simulink subsystem "Biblioteca_Iconos"  (R2023a)
settings: Solver=VariableStepAuto  StartTime=0.0  StopTime=10.0  RelTol=1e-3
undefined symbols (not defined in the file): baseRobot, baseRobot_, CdG, color, Icono, M, MdI, q0_, TabAje, X, Y, Z
libraries: sm_lib x1858, nesl_utility x164
(part 1 of 39)
settings Model: Creator=albher  LastModifiedBy=albher
settings SolverCC: AlgebraicLoopSolver=TrustRegion
settings DebuggingCC: UnconnectedInputMsg=warning  UnconnectedOutputMsg=warning  UnconnectedLineMsg=warning
settings ModelReferenceCC: EnableRefExpFcnMdlSchedulingChecks=on
settings RTWCC: DLArmComputeVersion=19.05

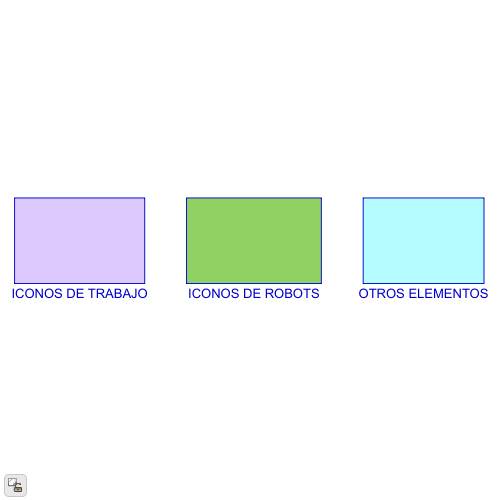
[thumbnail: Simulink's stored preview of the top-level diagram]
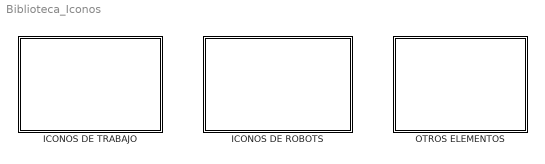
== system Biblioteca_Iconos ==
  ICONOS DE ROBOTS : Subsystem
  ICONOS DE TRABAJO : Subsystem
  OTROS ELEMENTOS : Subsystem

== system Biblioteca_Iconos/ICONOS DE ROBOTS ==
  note: image(imread(['auxStl/',tool.vNombre,'.png']))
  AbbIrb120_T_q : Subsystem  mask{base=baseRobot, q0=q0_}
      mask prompts: base "Base (x,y,z,Rz,Ry,Rx)"
      mask Display: image(imread('Robots/ABB_Irb120/AbbIrb120.png'))
  BrazoRobot : Subsystem  mask{base=baseRobot, q0=q0_}
      mask prompts: base "Base (x,y,z,Rz,Ry,Rx)"
      mask Display: image(imread('Robots/Rob_BrazoRobot/BrazoRobot.png'))
  Gofa : Subsystem  mask{base=baseRobot, q0=q0_}
      mask prompts: base "Base (x,y,z,Rz,Ry,Rx)"
      mask Display: image(imread('Robots/ABB_Gofa/abbGofa.png'))
  Humanoide : Subsystem  mask{base=baseRobot, q0=q0_}
      mask prompts: base "Base (x,y,z,Rz,Ry,Rx)"
      mask Display: image(imread('Robots/HUM_humanoide/humanoide.png'))
  Humanoide Brazos : Subsystem  mask{base=baseRobot, q0=q0_}
      mask prompts: base "Base (x,y,z,Rz,Ry,Rx)"
      mask Display: image(imread('Robots/HUM_humanoide/humanoide.png'))
  Humanoide de Pie : Subsystem  mask{base=baseRobot_, q0=q0_}
      mask prompts: base "Base (x,y,z,Rz,Ry,Rx)"
      mask Display: image(imread('Robots/HUM_humanoide/humanoide.png'))
  Niryo_Ned : Subsystem  mask{base=baseRobot, q0=q0_}
      mask prompts: base "Base(x,y,z,Rz,Ry,Rx)"
      mask Display: image(imread('Robots/NIRYO_niryo_ned/niryo_ned.png'))
  Poppy : Subsystem  mask{base=baseRobot, q0=q0_}
      mask prompts: base "Base (x,y,z,Rz,Ry,Rx)"
      mask Display: image(imread('./Robots/Poppy/Poppy.png'))
  TX40DH (q) : Subsystem  mask{base=baseRobot_, q0=q0_}
      mask prompts: base "Base [x,y,z,Rz,Ry,Rx]"
      mask init:
      | % DH de los ejes 1-6 no base
      | DH= [0, -pi/2, pi, 0, 0, 0;
      |      0.32, 0.035, 0, 0.225, 0, 0.065;
      |      0, 0.255, 0, 0, 0, 0;
      |      -pi/2, 0, pi/2, -pi/2, pi/2, 0];
      |  
      | % Sin incluir la base 
      | M= [10.8, 5.4, 4.05, 3.24, 2.16, 1.36];
      | 
      | CdG= [0, 0, 0, 0, 0, 0;
      |       0,  0, 0, 0, 0.05, 0;
      |       0.15, 0.2, 0, 0.05, 0, 0.03];
      | 
      |          % Ixx Iyy Izz Ixy Iyz Ixz
      | 
      | I=[0   ,    0.35,	0   ,	0,  0,	0;
      |    0.13 ,   0.524,	0.539,	0,	0,	0;
      |    0.066 ,  0.086,	0.0125,	0,	0,	0;
      |    0.0018,	0.0013,	0.0018,	0,	0,	0;
      |    3e-4,	4e-4,	3e-4,	0,	0,	0;
      |    1.5e-4,	1.5e-4,	4e-5,	0,	0,	0];
      | 
      | 
      | 
      | %limites
      | limits=[-pi, pi;  %Axis 1, minimum, maximum
      |         -2.18, 2.18;  %Axis 2, minimum, maximum
      |          -2.41, 2.41;   %Axis 3, minimum, maximum
      |         -4.71, 4.71;  %Axis 4, minimum, maximum
      |         -2.09, 2.09;  %Axis 5, minimum, maximum
      |         -4.71, 4.71]; %Axis 6, minimum, maximum
      |          
      | color= [1, 0.9, 0.15, 1];
      mask Display: image(imread('Robots/TX40/TX40.png'))
  "Tx90DH (q) " : Subsystem  mask{base=baseRobot_, q0=q0_}
      mask prompts: base "Base [x,y,z,Rz,Ry,Rx]"
      mask init:
      | % DH de los ejes 1-6 no base
      | DH= [0, -pi/2, pi, 0, 0, 0;
      |      0.478, 0.05, 0, 0.425, 0, 0.1;
      |      0.05, 0.425, 0, 0, 0, 0;
      |      -pi/2, 0, pi/2, -pi/2, pi/2, 0];
      |  
      | % Sin incluir la base 
      | M= [34.73, 39.27, 15.13, 21.25, 0.42, 0.03];
      | 
      | CdG= [-0.13, 0, 0.05, 0, 0.01, 0;
      |       0.47,  0, -0.55, 0.004, 0, 0;
      |       -0.18, 0, -0.14, 0, 0, 0];
      | 
      |          % Ixx Iyy Izz Ixy Iyz Ixz
      | I=[0   ,    0.35,	0   ,	0,  0,	0;
      |    0.13 ,   0.524,	0.539,	0,	0,	0;
      |    0.066 ,  0.086,	0.0125,	0,	0,	0;
      |    0.0018,	0.0013,	0.0018,	0,	0,	0;
      |    3e-4,	4e-4,	3e-4,	0,	0,	0;
      |    1.5e-4,	1.5e-4,	4e-5,	0,	0,	0];
      | 
      | %limites
      | limits=[-pi, pi;  %Axis 1, minimum, maximum
      |         -2.27, 2.57;  %Axis 2, minimum, maximum
      |         -2.53, 2.53;   %Axis 3, minimum, maximum
      |         -4.71, 4.71;  %Axis 4, minimum, maximum
      |         -2.007, 2.443;  %Axis 5, minimum, maximum
      |         -4.71, 4.71]; %Axis 6, minimum, maximum
      |          
      | color= [1, 0.4, 0.5, 1];
      mask Display: image(imread('Robots/TX90/TX90.png'))
  UR10_DH : Subsystem  mask{base=baseRobot_, q0=q0_}
      mask prompts: base "Base [x,y,z,Rz,Ry,Rx]"
      mask init:
      | % DH de los ejes 1-6 no base
      | DH= [0, pi/2, 0, -pi/2, 0, 0;
      |      0.128, 0.176, -0.128, 0.116, 0.116, 0.092;
      |      0, 0.612, 0.572, 0, 0, 0;
      |      pi/2, 0, 0, -pi/2, pi/2, 0];
      |  
      | % Sin incluir la base 
      | M= [25, 27, 15, 10, 2.5, 1.5];
      | 
      | CdG= [0, -0.05, -0.0203, 0, 0, 0;
      |       0,  0.006, -0.0141, 0.019, 0, 0;
      |       0, 0.1, 0.070, 0, 0, 0.032];
      | 
      |          % Ixx Iyy Izz Ixy Iyz Ixz
      | I=[0   ,    0.35,	0   ,	0,  0,	0;
      |    0.13 ,   0.524,	0.539,	0,	0,	0;
      |    0.066 ,  0.086,	0.0125,	0,	0,	0;
      |    0.0018,	0.0013,	0.0018,	0,	0,	0;
      |    3e-4,	4e-4,	3e-3,	0,	0,	0;
      |    1.5e-4,	1.5e-4,	4e-3,	0,	0,	0];
      | 
      | %limites
      | limits=[-pi, pi;  %Axis 1, minimum, maximum
      |         -1.74, 1.74;  %Axis 2, minimum, maximum
      |          -3.84, 3.84;   %Axis 3, minimum, maximum
      |         -3.49, 3.49;  %Axis 4, minimum, maximum
      |         -2.09, 2.09;  %Axis 5, minimum, maximum
      |         -6.98, 6.98]; %Axis 6, minimum, maximum
      |          
      | color= [0.4, 0.4, 0.6, 1];
      mask Display: image(imread('Robots/UR_UR10_DH/UR10.png'))
  gripper_3f : Subsystem  mask{base=baseRobot, q0=q0_}
      mask prompts: base "Base (x,y,z,Rz,Ry,Rx)"
      mask Display: image(imread('./Robots/gripper_3f/gripper_3f.png'))
  irb120 : Subsystem  mask{base=baseRobot, q0=q0_}
      mask prompts: base "Base (x,y,z,Rz,Ry,Rx)"
      mask Display: image(imread('Robots/ABB_irb120/AbbIrb120.png'))
  irb120_DH : Subsystem  mask{base=baseRobot, q0=q0_}
      mask prompts: base "Base [x,y,z,Rz,Ry,Rx]"
      mask init:
      | % DH de los ejes 1-6 no base
      | DH= [0, -pi/2, 0, 0, 0, pi;
      |      0.290, 0, 0, 0.302, 0, 0.072;
      |      0, 0.270, 0.070, 0, 0, 0;
      |      -pi/2, 0, -pi/2, pi/2, -pi/2, 0];
      | % Dinámica del sistema. Includo la base
      | M= 1*ones(1,7);
      | CdG= zeros(3,7);
      | MdI= 0.01*ones(6,7);
      | color= [1, 0.43, 0, 1];
      | 
      | % Límite de los ejes (rad)
      | Lim= [-165, -110, -110, -160, -120, -400;
      |       165,   110,  70,   160,  120,  400]*pi/180;
      mask Display: image(imread('Robots/ABB_irb120_DH/irb120DH.png'))
  kinovaJaco : Subsystem  mask{base=baseRobot, q0=q0_}
      mask prompts: base "Base(x,y,z,Rz,Ry,Rx)"
      mask Display: image(imread('Robots/KIN_kinova2Arm/kinovaJaco.png'))
  "puma560_DH " : Subsystem  mask{base=baseRobot, q0=q0_}
      mask prompts: base "Base [x,y,z,Rz,Ry,Rx]"
      mask init:
      | % DH de los ejes 1-6 no base
      | DH= [0, 0, 0, 0, 0, 0;
      |      0, 0, 0.15005, 0.4318, 0, 0.0;
      |      0, 0.4318, 0.0203, 0, 0, 0;
      |      pi/2, 0, -pi/2, pi/2, -pi/2, 0];
      |  
      | % Sin incluir la base 
      | M= [0, 17.4, 4.8, 0.82, 0.34, 0.09];
      | 
      | CdG= [0, -0.3638, -0.0203, 0, 0, 0;
      |       0,  0.006, -0.0141, 0.019, 0, 0;
      |       0, 0.2275, 0.070, 0, 0, 0];
      | 
      |          % Ixx Iyy Izz Ixy Iyz Ixz
      | I=[0   ,    0.35,	0   ,	0,  0,	0;
      |    0.13 ,   0.524,	0.539,	0,	0,	0;
      |    0.066 ,  0.086,	0.0125,	0,	0,	0;
      |    0.0018,	0.0013,	0.0018,	0,	0,	0;
      |    3e-4,	4e-4,	3e-4,	0,	0,	0;
      |    1.5e-4,	1.5e-4,	4e-5,	0,	0,	0];
      | 
      | %limites
      | limits=[-2.79, 2.79;  %Axis 1, minimum, maximum
      |         -1.92, 1.92;  %Axis 2, minimum, maximum
      |          -2.356, 2.356;   %Axis 3, minimum, maximum
      |         -4.642, 4.642;  %Axis 4, minimum, maximum
      |         -1.745, 1.745;  %Axis 5, minimum, maximum
      |         -4.642, 4.642]; %Axis 6, minimum, maximum
      |          
      | color= [0.4, 0.8, 0.51, 1];
      mask Display: image(imread('Robots/UNI_puma560_DH/puma560.png'))
  sawyerDH (q) : Subsystem  mask{base=baseRobot, q0=q0_}
      mask prompts: base "Base [x,y,z,Rz,Ry,Rx]"
      mask init:
      | % DH de los ejes 1-6 no base
      | DH= [0, -pi/2, 0, 0, 0, 0, 0;
      |      0.317, 0.1925, 0.4, -0.1685, 0.4, 0.1363, 0.13375;
      |      0.081, 0.0, 0.0, 0.0, 0, 0, 0;
      |      -pi/2, -pi/2, pi/2, -pi/2, pi/2, -pi/2, 0];
      |  
      | % Sin incluir la base 
      | M= [25, 27, 15, 10, 2.5,1.5, 0.09];
      | 
      | CdG= [0, -0.05, -0.0203, 0, 0, 0,0;
      |       0,  0.006, -0.0141, 0.019, 0, 0,0;
      |       0, 0.1, 0.070, 0, 0, 0.032,0];
      | 
      |          % Ixx Iyy Izz Ixy Iyz Ixz
      | I=[0   ,    0.35,	0   ,	0,  0,	0;
      |    0.13 ,   0.524,	0.539,	0,	0,	0;
      |    0.066 ,  0.086,	0.0125,	0,	0,	0;
      |    0.0018,	0.0013,	0.0018,	0,	0,	0;
      |    3e-4,	4e-4,	3e-4,	0,	0,	0;
      |    1.5e-4,	1.5e-4,	4e-5,	0,	0,	0;
      |    1.5e-4,	1.5e-4,	4e-5,	0,	0,	0];
      | 
      | %limites
      | limits=[-pi, pi;  %Axis 1, minimum, maximum
      |         -1.745, 1.745;  %Axis 2, minimum, maximum
      |         -3.84, 3.84;   %Axis 3, minimum, maximum
      |         -3.49, 3.49;  %Axis 4, minimum, maximum
      |         -2.094, 2.094;  %Axis 5, minimum, maximum
      |         -6.98, 6.98; %Axis 6, minimum, maximum
      |         -6.98, 6.98]; %Axis 7, minimum, maximum
      |         
      | color= [1, 0.18, 0.2, 1];
      mask Display: image(imread('Robots/SAWYER/SAWYER.png'))

== system Biblioteca_Iconos/ICONOS DE TRABAJO ==
  "Icono Variable Terminal " : Subsystem  mask{tool=Icono}
      mask prompts: tool "Struct(base, tcp, masa, cdg, inercia)"
      mask init:
      | % Esta zona se ejecuta antes de la simulación
      |  % Nombre de modelo y del bloque
      |  modelo= get_param(0 ,'CurrentSystem');
      |  block= get_param(modelo,'CurrentBlock');
      |  % Path del icono visual
      |  path=[modelo,'/',block,'/Visual'];
      |  % Propiedad del nombre del fichero externo a introducir
      |  get_param(path, 'ExtGeomFileName');
      |  % Poner el nombre del objeto pieza
      |  set_param(path,'ExtGeomFileName',['Biblioteca/',tool.nombre,'.stl']);
      |  % get_param(path, 'ExtGeomFileName')
      |  % image(imread(['Biblioteca/',tool.nombre,'.png']))
      mask Display:
      | % Esta zona se ejecuta después de ñla simulación
      | 
      | % tool.nombre
      | %  modelo= get_param(0 ,'CurrentSystem')
      | %  block= get_param(modelo,'CurrentBlock')
      | %  path=[modelo,'/',block,'/Visual']
      | %  get_param(path, 'ExtGeomFileName')
      | %  set_param(path,'ExtGeomFileName',['Biblioteca/',tool.nombre,'.stl'])
      | %  get_param(path, 'ExtGeomFileName')
      | 
      | % Icono de la mascara
      | image(imread(['Biblioteca/',tool.nombre,'.png']));
  Icono Variable con Eje fijo : Subsystem  mask{tool=Icono}
      mask prompts: tool "Struct(base, tcp, masa, cdg, inercia)"
      mask init: same as Biblioteca_Iconos/ICONOS DE TRABAJO/Icono Variable Terminal 
      mask Display:
      | % Esta zona se ejecuta después de ñla simulación
      | 
      | % tool.nombre
      | %  modelo= get_param(0 ,'CurrentSystem')
      | %  block= get_param(modelo,'CurrentBlock')
      | %  path=[modelo,'/',block,'/Visual']
      | %  get_param(path, 'ExtGeomFileName')
      | %  set_param(path,'ExtGeomFileName',['Biblioteca/',tool.nombre,'.stl'])
      | %  get_param(path, 'ExtGeomFileName')
      | 
      | % Icono de la mascara
      | image(imread(['Biblioteca/',tool.nombre,'.png']));
  TabAje : Subsystem  mask{tool=TabAje}
      mask prompts: tool "Struct(base, tcp, masa, cdg, inercia)"
      mask Display:
      | %disp('Pinza')
      | image(imread(['Biblioteca/TabAjedrez.png']))

== system Biblioteca_Iconos/OTROS ELEMENTOS ==
  Infinite Plane : sm_lib/Curves and Surfaces/Infinite Plane  GraphicType=Rectangle  GraphicPlaneWidth=1  GraphicPlaneWidthUnits=m  GraphicPlaneHeight=1  GraphicPlaneHeightUnits=m  GraphicVisPropType=SimpleVisualProperties  GraphicDiffuseColor=[0.5 0.5 0.5]  GraphicOpacity=0.25  GraphicSpecularColor=[0.5 0.5 0.5 1.0]  GraphicAmbientColor=[0.15 0.15 0.15 1.0]  GraphicEmissiveColor=[0.0 0.0 0.0 1.0]  GraphicShininess=75
  Link_Basico : Subsystem
  MechanismConfiguration : sm_lib/Utilities/Mechanism Configuration  UniformGravity=Constant  GravityVector=[0 0 -9.80665]  GravityVectorUnits=m/s^2  LinearizationDelta=0.001  JointModeTransitionNonlinearIterations=2
  Prismatic Joint : sm_lib/Joints/Prismatic Joint  JointMode=Normal  SenseConstraintForce=off  SenseConstraintForceX=off  SenseConstraintForceY=off  SenseConstraintForceZ=off  SenseConstraintTorque=off  SenseConstraintTorqueX=off  SenseConstraintTorqueY=off  SenseConstraintTorqueZ=off  SenseTotalForce=off  SenseTotalForceX=off  SenseTotalForceY=off  SenseTotalForceZ=off  SenseTotalTorque=off  SenseTotalTorqueX=off  SenseTotalTorqueY=off  SenseTotalTorqueZ=off  CompositeWrenchDir=FollowerOnBase  CompositeWrenchFrame=BaseFrame  EquilibriumPosition=0  EquilibriumPositionUnits=m  SpringStiffness=0  SpringStiffnessUnits=N/m  DampingCoefficient=0  DampingCoefficientUnits=N/(m/s)  TorqueActuationMode=NoTorque  MotionActuationMode=ComputedMotion  SensePosition=off  SenseVelocity=off  SenseAcceleration=off  SenseTorqueForce=off  SenseLowerLimitTorqueForce=off  SenseUpperLimitTorqueForce=off  LowerLimitSpecify=off  LowerLimitBound=-1  LowerLimitBoundUnits=m  LowerLimitStiffness=1e6  LowerLimitStiffnessUnits=N/m  LowerLimitDamping=1e3  LowerLimitDampingUnits=N/(m/s)  LowerLimitTransitionRegionWidth=1e-4  LowerLimitTransitionRegionWidthUnits=m  UpperLimitSpecify=off  UpperLimitBound=1  UpperLimitBoundUnits=m  UpperLimitStiffness=1e6  UpperLimitStiffnessUnits=N/m  UpperLimitDamping=1e3  UpperLimitDampingUnits=N/(m/s)  UpperLimitTransitionRegionWidth=1e-4  UpperLimitTransitionRegionWidthUnits=m  PositionTargetSpecify=off  PositionTargetPriority=High  PositionTargetValue=0  PositionTargetValueUnits=m  VelocityTargetSpecify=off  VelocityTargetPriority=High  VelocityTargetValue=0  VelocityTargetValueUnits=m/s
  Reference Frame : sm_lib/Frames and Transforms/Reference Frame
  Revolute Joint : sm_lib/Joints/Revolute Joint  JointMode=Normal  SenseConstraintForce=off  SenseConstraintForceX=off  SenseConstraintForceY=off  SenseConstraintForceZ=off  SenseConstraintTorque=off  SenseConstraintTorqueX=off  SenseConstraintTorqueY=off  SenseConstraintTorqueZ=off  SenseTotalForce=off  SenseTotalForceX=off  SenseTotalForceY=off  SenseTotalForceZ=off  SenseTotalTorque=off  SenseTotalTorqueX=off  SenseTotalTorqueY=off  SenseTotalTorqueZ=off  CompositeWrenchDir=FollowerOnBase  CompositeWrenchFrame=BaseFrame  EquilibriumPosition=0  EquilibriumPositionUnits=deg  SpringStiffness=0  SpringStiffnessUnits=N*m/deg  DampingCoefficient=0  DampingCoefficientUnits=N*m/(deg/s)  TorqueActuationMode=NoTorque  MotionActuationMode=ComputedMotion  SensePosition=off  SenseVelocity=off  SenseAcceleration=off  SenseTorqueForce=off  SenseLowerLimitTorqueForce=off  SenseUpperLimitTorqueForce=off  LowerLimitSpecify=off  LowerLimitBound=-90  LowerLimitBoundUnits=deg  LowerLimitStiffness=1e4  LowerLimitStiffnessUnits=N*m/deg  LowerLimitDamping=10  LowerLimitDampingUnits=N*m/(deg/s)  LowerLimitTransitionRegionWidth=0.1  LowerLimitTransitionRegionWidthUnits=deg  UpperLimitSpecify=off  UpperLimitBound=90  UpperLimitBoundUnits=deg  UpperLimitStiffness=1e4  UpperLimitStiffnessUnits=N*m/deg  UpperLimitDamping=10  UpperLimitDampingUnits=N*m/(deg/s)  UpperLimitTransitionRegionWidth=0.1  UpperLimitTransitionRegionWidthUnits=deg  PositionTargetSpecify=off  PositionTargetPriority=High  PositionTargetValue=0  PositionTargetValueUnits=deg  VelocityTargetSpecify=off  VelocityTargetPriority=High  VelocityTargetValue=0  VelocityTargetValueUnits=deg/s
  Solver Configuration : nesl_utility/Solver Configuration  PhysicalDomain=network_engine_domain  SubClassName=solver  LeftPortType=input  RightPortType=generic  Tones=[]  Harmonics=[]  SimulateNoise=off  Profile=off  UseLocalSampling=off  EnableSwitchedLinearOptims=on  FrequencyDomain=off  UseCCode=off  RelTol=0.001  AbsTol=1e-06  MinStep=1e-09  ToWorkspace=off  RevertToSquareIcSolve=off  NumHomotopyIterations=100  PhasorMode=off  PhasorModeNumHarmonics=1  ConsistencySolver=NEWTON_FTOL  IndexReductionMethod=DerivativeReplacement  DoDC=off  ResidualTolerance=1e-09  ConsistencyTolSource=GLOBAL  ConsistencyAbsTol=0.001  ConsistencyRelTol=0.001  ConsistencyTolFactor=0.001  UseLocalSolver=off  LocalSolverChoice=NE_BACKWARD_EULER_ADVANCER  ResolveIndetEquations=on  FunctionEvalNumThread=1  LocalSolverSampleTime=0.001  DoFixedCost=off  MaxNonlinIter=3  MaxModeIter=2  ComputeImpulses=off  ImpulseIterations=2  LinearAlgebra=auto  LinearAlgebraNumThread=0  EquationFormulation=NE_TIME_EF  DelaysMemoryBudget=1024  AutomaticFiltering=on  FilteringTimeConstant=0.001  PartitionStorageMethod=AS_NEEDED  PartitionMemoryBudget=1024  PartitionMethod=ROBUST
  Spline : sm_lib/Curves and Surfaces/Spline  GraphicAmbientColor=[0.15 0.15 0.15 1.0]  GraphicDiffuseColor=[0.0 0.0 0.0]  DataPoints=pose  DataPointsUnits=m  GraphicEmissiveColor=[0.0 0.0 0.0 1.0]  EndConditionType=Natural  MarkerShape=Frame  MarkerSize=10  GraphicType=FromGeometry  GraphicOpacity=1.0  GraphicShininess=75  GraphicSpecularColor=[0.5 0.5 0.5 1.0]  GraphicVisPropType=SimpleVisualProperties
  Weld Joint : sm_lib/Joints/Weld Joint  JointMode=Normal  SenseConstraintForce=off  SenseConstraintForceX=off  SenseConstraintForceY=off  SenseConstraintForceZ=off  SenseConstraintTorque=off  SenseConstraintTorqueX=off  SenseConstraintTorqueY=off  SenseConstraintTorqueZ=off  SenseTotalForce=off  SenseTotalForceX=off  SenseTotalForceY=off  SenseTotalForceZ=off  SenseTotalTorque=off  SenseTotalTorqueX=off  SenseTotalTorqueY=off  SenseTotalTorqueZ=off  CompositeWrenchDir=FollowerOnBase  CompositeWrenchFrame=BaseFrame
  World : sm_lib/Frames and Transforms/World Frame

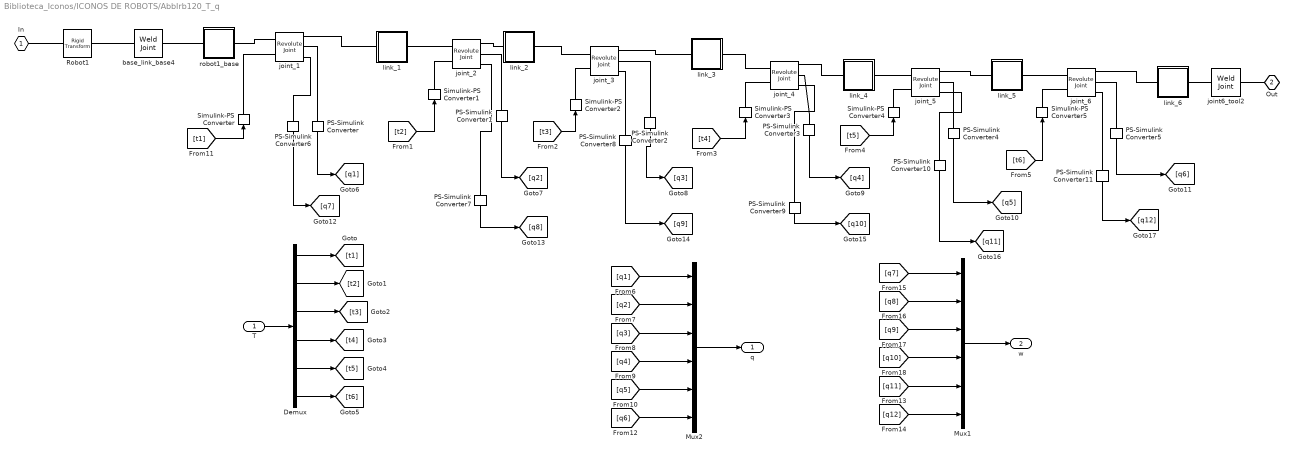
== system Biblioteca_Iconos/ICONOS DE ROBOTS/AbbIrb120_T_q ==
  T : Inport
  Demux : Demux  Outputs=6
  Mux1 : Mux  Inputs=6
  Mux2 : Mux  Inputs=6
  PS-Simulink Converter{,1..11} (12 alike) : nesl_utility/PS-Simulink Converter  PhysicalDomain=network_engine_domain  SubClassName=ps_output  LeftPortType=input  RightPortType=output  PseudoPeriodic=off  Frequencies=[]  VectorFormat=1-D array  Unit=inherit  AffineConversion=off
  Robot1 : sm_lib/Frames and Transforms/Rigid Transform  TranslationMethod=Cartesian  TranslationStandardOffset=0  TranslationStandardOffsetUnits=m  TranslationStandardAxis=+Z  TranslationCartesianOffset=base(1:3)  TranslationCartesianOffsetUnits=m  TranslationROffset=0  TranslationROffsetUnits=m  TranslationZOffset=0  TranslationZOffsetUnits=m  TranslationThetaOffset=0  TranslationThetaOffsetUnits=deg  RotationMethod=RotationSequence  RotationAngleUnits=deg  RotationStandardAxis=+Z  RotationAngle=0.0  RotationArbitraryAxis=[0 0 1]  FollAlignAxisA=+X  BaseAlignAxisA=+Y  FollAlignAxisB=+Y  BaseAlignAxisB=+Z  RotationSequenceAxes=FollowerAxes  RotationSequence=ZYX  RotationSequenceAngles=base(4:6)  RotationSequenceAnglesUnits=rad  RotationMatrix=[1 0 0; 0 1 0; 0 0 1]  Quaternion=[1 0 0 0]
  Simulink-PS Converter{,1..5} (6 alike) : nesl_utility/Simulink-PS Converter  PhysicalDomain=network_engine_domain  SubClassName=ps_input  LeftPortType=input  RightPortType=output  PseudoPeriodic=off  Frequencies=[]  NoiseDistribution=none  NoiseParameters=[]  Unit=1  AffineConversion=off  FilteringAndDerivatives=provide  SimscapeFilterOrder=1  InputFilterTimeConstant=0.001  UdotUserProvided=0
  base_link_base4 : sm_lib/Joints/Weld Joint  JointMode=Normal  SenseConstraintForce=off  SenseConstraintForceX=off  SenseConstraintForceY=off  SenseConstraintForceZ=off  SenseConstraintTorque=off  SenseConstraintTorqueX=off  SenseConstraintTorqueY=off  SenseConstraintTorqueZ=off  SenseTotalForce=off  SenseTotalForceX=off  SenseTotalForceY=off  SenseTotalForceZ=off  SenseTotalTorque=off  SenseTotalTorqueX=off  SenseTotalTorqueY=off  SenseTotalTorqueZ=off  CompositeWrenchDir=FollowerOnBase  CompositeWrenchFrame=BaseFrame
  joint6_tool2 : sm_lib/Joints/Weld Joint  JointMode=Normal  SenseConstraintForce=off  SenseConstraintForceX=off  SenseConstraintForceY=off  SenseConstraintForceZ=off  SenseConstraintTorque=off  SenseConstraintTorqueX=off  SenseConstraintTorqueY=off  SenseConstraintTorqueZ=off  SenseTotalForce=off  SenseTotalForceX=off  SenseTotalForceY=off  SenseTotalForceZ=off  SenseTotalTorque=off  SenseTotalTorqueX=off  SenseTotalTorqueY=off  SenseTotalTorqueZ=off  CompositeWrenchDir=FollowerOnBase  CompositeWrenchFrame=BaseFrame
  joint_1 : sm_lib/Joints/Revolute Joint  JointMode=Normal  SenseConstraintForce=off  SenseConstraintForceX=off  SenseConstraintForceY=off  SenseConstraintForceZ=off  SenseConstraintTorque=off  SenseConstraintTorqueX=off  SenseConstraintTorqueY=off  SenseConstraintTorqueZ=off  SenseTotalForce=off  SenseTotalForceX=off  SenseTotalForceY=off  SenseTotalForceZ=off  SenseTotalTorque=off  SenseTotalTorqueX=off  SenseTotalTorqueY=off  SenseTotalTorqueZ=off  CompositeWrenchDir=FollowerOnBase  CompositeWrenchFrame=BaseFrame  EquilibriumPosition=0  EquilibriumPositionUnits=deg  SpringStiffness=0  SpringStiffnessUnits=N*m/deg  DampingCoefficient=0  DampingCoefficientUnits=m^2*kg/s/rad  TorqueActuationMode=InputTorque  MotionActuationMode=ComputedMotion  SensePosition=on  SenseVelocity=on  SenseAcceleration=off  SenseTorqueForce=off  SenseLowerLimitTorqueForce=off  SenseUpperLimitTorqueForce=off  LowerLimitSpecify=on  LowerLimitBound=-2.87979  LowerLimitBoundUnits=rad  LowerLimitStiffness=1e4  LowerLimitStiffnessUnits=N*m/deg  LowerLimitDamping=10  LowerLimitDampingUnits=N*m/(deg/s)  LowerLimitTransitionRegionWidth=0.1  LowerLimitTransitionRegionWidthUnits=deg  UpperLimitSpecify=on  UpperLimitBound=2.87979  UpperLimitBoundUnits=rad  UpperLimitStiffness=1e4  UpperLimitStiffnessUnits=N*m/deg  UpperLimitDamping=10  UpperLimitDampingUnits=N*m/(deg/s)  UpperLimitTransitionRegionWidth=0.1  UpperLimitTransitionRegionWidthUnits=deg  PositionTargetSpecify=on  PositionTargetPriority=High  PositionTargetValue=q0(1)  PositionTargetValueUnits=rad  VelocityTargetSpecify=off  VelocityTargetPriority=High  VelocityTargetValue=0  VelocityTargetValueUnits=deg/s
  joint_2 : sm_lib/Joints/Revolute Joint  JointMode=Normal  SenseConstraintForce=off  SenseConstraintForceX=off  SenseConstraintForceY=off  SenseConstraintForceZ=off  SenseConstraintTorque=off  SenseConstraintTorqueX=off  SenseConstraintTorqueY=off  SenseConstraintTorqueZ=off  SenseTotalForce=off  SenseTotalForceX=off  SenseTotalForceY=off  SenseTotalForceZ=off  SenseTotalTorque=off  SenseTotalTorqueX=off  SenseTotalTorqueY=off  SenseTotalTorqueZ=off  CompositeWrenchDir=FollowerOnBase  CompositeWrenchFrame=BaseFrame  EquilibriumPosition=0  EquilibriumPositionUnits=deg  SpringStiffness=0  SpringStiffnessUnits=N*m/deg  DampingCoefficient=0  DampingCoefficientUnits=m^2*kg/s/rad  TorqueActuationMode=InputTorque  MotionActuationMode=ComputedMotion  SensePosition=on  SenseVelocity=on  SenseAcceleration=off  SenseTorqueForce=off  SenseLowerLimitTorqueForce=off  SenseUpperLimitTorqueForce=off  LowerLimitSpecify=on  LowerLimitBound=-1.91986  LowerLimitBoundUnits=rad  LowerLimitStiffness=1e4  LowerLimitStiffnessUnits=N*m/deg  LowerLimitDamping=10  LowerLimitDampingUnits=N*m/(deg/s)  LowerLimitTransitionRegionWidth=0.1  LowerLimitTransitionRegionWidthUnits=deg  UpperLimitSpecify=on  UpperLimitBound=1.91986  UpperLimitBoundUnits=rad  UpperLimitStiffness=1e4  UpperLimitStiffnessUnits=N*m/deg  UpperLimitDamping=10  UpperLimitDampingUnits=N*m/(deg/s)  UpperLimitTransitionRegionWidth=0.1  UpperLimitTransitionRegionWidthUnits=deg  PositionTargetSpecify=on  PositionTargetPriority=High  PositionTargetValue=q0(2)  PositionTargetValueUnits=rad  VelocityTargetSpecify=off  VelocityTargetPriority=High  VelocityTargetValue=0  VelocityTargetValueUnits=deg/s
  joint_3 : sm_lib/Joints/Revolute Joint  JointMode=Normal  SenseConstraintForce=off  SenseConstraintForceX=off  SenseConstraintForceY=off  SenseConstraintForceZ=off  SenseConstraintTorque=off  SenseConstraintTorqueX=off  SenseConstraintTorqueY=off  SenseConstraintTorqueZ=off  SenseTotalForce=off  SenseTotalForceX=off  SenseTotalForceY=off  SenseTotalForceZ=off  SenseTotalTorque=off  SenseTotalTorqueX=off  SenseTotalTorqueY=off  SenseTotalTorqueZ=off  CompositeWrenchDir=FollowerOnBase  CompositeWrenchFrame=BaseFrame  EquilibriumPosition=0  EquilibriumPositionUnits=deg  SpringStiffness=0  SpringStiffnessUnits=N*m/deg  DampingCoefficient=0  DampingCoefficientUnits=m^2*kg/s/rad  TorqueActuationMode=InputTorque  MotionActuationMode=ComputedMotion  SensePosition=on  SenseVelocity=on  SenseAcceleration=off  SenseTorqueForce=off  SenseLowerLimitTorqueForce=off  SenseUpperLimitTorqueForce=off  LowerLimitSpecify=on  LowerLimitBound=-1.91986  LowerLimitBoundUnits=rad  LowerLimitStiffness=1e4  LowerLimitStiffnessUnits=N*m/deg  LowerLimitDamping=10  LowerLimitDampingUnits=N*m/(deg/s)  LowerLimitTransitionRegionWidth=0.1  LowerLimitTransitionRegionWidthUnits=deg  UpperLimitSpecify=on  UpperLimitBound=1.22173  UpperLimitBoundUnits=rad  UpperLimitStiffness=1e4  UpperLimitStiffnessUnits=N*m/deg  UpperLimitDamping=10  UpperLimitDampingUnits=N*m/(deg/s)  UpperLimitTransitionRegionWidth=0.1  UpperLimitTransitionRegionWidthUnits=deg  PositionTargetSpecify=on  PositionTargetPriority=High  PositionTargetValue=q0(3)  PositionTargetValueUnits=rad  VelocityTargetSpecify=off  VelocityTargetPriority=High  VelocityTargetValue=0  VelocityTargetValueUnits=deg/s
  joint_4 : sm_lib/Joints/Revolute Joint  JointMode=Normal  SenseConstraintForce=off  SenseConstraintForceX=off  SenseConstraintForceY=off  SenseConstraintForceZ=off  SenseConstraintTorque=off  SenseConstraintTorqueX=off  SenseConstraintTorqueY=off  SenseConstraintTorqueZ=off  SenseTotalForce=off  SenseTotalForceX=off  SenseTotalForceY=off  SenseTotalForceZ=off  SenseTotalTorque=off  SenseTotalTorqueX=off  SenseTotalTorqueY=off  SenseTotalTorqueZ=off  CompositeWrenchDir=FollowerOnBase  CompositeWrenchFrame=BaseFrame  EquilibriumPosition=0  EquilibriumPositionUnits=deg  SpringStiffness=0  SpringStiffnessUnits=N*m/deg  DampingCoefficient=0  DampingCoefficientUnits=m^2*kg/s/rad  TorqueActuationMode=InputTorque  MotionActuationMode=ComputedMotion  SensePosition=on  SenseVelocity=on  SenseAcceleration=off  SenseTorqueForce=off  SenseLowerLimitTorqueForce=off  SenseUpperLimitTorqueForce=off  LowerLimitSpecify=on  LowerLimitBound=-2.79253  LowerLimitBoundUnits=rad  LowerLimitStiffness=1e4  LowerLimitStiffnessUnits=N*m/deg  LowerLimitDamping=10  LowerLimitDampingUnits=N*m/(deg/s)  LowerLimitTransitionRegionWidth=0.1  LowerLimitTransitionRegionWidthUnits=deg  UpperLimitSpecify=on  UpperLimitBound=2.79253  UpperLimitBoundUnits=rad  UpperLimitStiffness=1e4  UpperLimitStiffnessUnits=N*m/deg  UpperLimitDamping=10  UpperLimitDampingUnits=N*m/(deg/s)  UpperLimitTransitionRegionWidth=0.1  UpperLimitTransitionRegionWidthUnits=deg  PositionTargetSpecify=on  PositionTargetPriority=High  PositionTargetValue=q0(4)  PositionTargetValueUnits=rad  VelocityTargetSpecify=off  VelocityTargetPriority=High  VelocityTargetValue=0  VelocityTargetValueUnits=deg/s
  joint_5 : sm_lib/Joints/Revolute Joint  JointMode=Normal  SenseConstraintForce=off  SenseConstraintForceX=off  SenseConstraintForceY=off  SenseConstraintForceZ=off  SenseConstraintTorque=off  SenseConstraintTorqueX=off  SenseConstraintTorqueY=off  SenseConstraintTorqueZ=off  SenseTotalForce=off  SenseTotalForceX=off  SenseTotalForceY=off  SenseTotalForceZ=off  SenseTotalTorque=off  SenseTotalTorqueX=off  SenseTotalTorqueY=off  SenseTotalTorqueZ=off  CompositeWrenchDir=FollowerOnBase  CompositeWrenchFrame=BaseFrame  EquilibriumPosition=0  EquilibriumPositionUnits=deg  SpringStiffness=0  SpringStiffnessUnits=N*m/deg  DampingCoefficient=0  DampingCoefficientUnits=m^2*kg/s/rad  TorqueActuationMode=InputTorque  MotionActuationMode=ComputedMotion  SensePosition=on  SenseVelocity=on  SenseAcceleration=off  SenseTorqueForce=off  SenseLowerLimitTorqueForce=off  SenseUpperLimitTorqueForce=off  LowerLimitSpecify=on  LowerLimitBound=-2.094395  LowerLimitBoundUnits=rad  LowerLimitStiffness=1e4  LowerLimitStiffnessUnits=N*m/deg  LowerLimitDamping=10  LowerLimitDampingUnits=N*m/(deg/s)  LowerLimitTransitionRegionWidth=0.1  LowerLimitTransitionRegionWidthUnits=deg  UpperLimitSpecify=on  UpperLimitBound=2.094395  UpperLimitBoundUnits=rad  UpperLimitStiffness=1e4  UpperLimitStiffnessUnits=N*m/deg  UpperLimitDamping=10  UpperLimitDampingUnits=N*m/(deg/s)  UpperLimitTransitionRegionWidth=0.1  UpperLimitTransitionRegionWidthUnits=deg  PositionTargetSpecify=on  PositionTargetPriority=High  PositionTargetValue=q0(5)  PositionTargetValueUnits=rad  VelocityTargetSpecify=off  VelocityTargetPriority=High  VelocityTargetValue=0  VelocityTargetValueUnits=deg/s
  joint_6 : sm_lib/Joints/Revolute Joint  JointMode=Normal  SenseConstraintForce=off  SenseConstraintForceX=off  SenseConstraintForceY=off  SenseConstraintForceZ=off  SenseConstraintTorque=off  SenseConstraintTorqueX=off  SenseConstraintTorqueY=off  SenseConstraintTorqueZ=off  SenseTotalForce=off  SenseTotalForceX=off  SenseTotalForceY=off  SenseTotalForceZ=off  SenseTotalTorque=off  SenseTotalTorqueX=off  SenseTotalTorqueY=off  SenseTotalTorqueZ=off  CompositeWrenchDir=FollowerOnBase  CompositeWrenchFrame=BaseFrame  EquilibriumPosition=0  EquilibriumPositionUnits=deg  SpringStiffness=0  SpringStiffnessUnits=N*m/deg  DampingCoefficient=0  DampingCoefficientUnits=m^2*kg/s/rad  TorqueActuationMode=InputTorque  MotionActuationMode=ComputedMotion  SensePosition=on  SenseVelocity=on  SenseAcceleration=off  SenseTorqueForce=off  SenseLowerLimitTorqueForce=off  SenseUpperLimitTorqueForce=off  LowerLimitSpecify=on  LowerLimitBound=-6.98132  LowerLimitBoundUnits=rad  LowerLimitStiffness=1e4  LowerLimitStiffnessUnits=N*m/deg  LowerLimitDamping=10  LowerLimitDampingUnits=N*m/(deg/s)  LowerLimitTransitionRegionWidth=0.1  LowerLimitTransitionRegionWidthUnits=deg  UpperLimitSpecify=on  UpperLimitBound=6.98132  UpperLimitBoundUnits=rad  UpperLimitStiffness=1e4  UpperLimitStiffnessUnits=N*m/deg  UpperLimitDamping=10  UpperLimitDampingUnits=N*m/(deg/s)  UpperLimitTransitionRegionWidth=0.1  UpperLimitTransitionRegionWidthUnits=deg  PositionTargetSpecify=on  PositionTargetPriority=High  PositionTargetValue=q0(6)  PositionTargetValueUnits=rad  VelocityTargetSpecify=off  VelocityTargetPriority=High  VelocityTargetValue=0  VelocityTargetValueUnits=deg/s
  link_1 : Subsystem
  link_2 : Subsystem
  link_3 : Subsystem
  link_4 : Subsystem
  link_5 : Subsystem
  link_6 : Subsystem
  robot1_base : Subsystem
  In : PMIOPort  Side=Left
  Out : PMIOPort  Port=2  Side=Right
  q : Outport  VectorParamsAs1DForOutWhenUnconnected=off
  w : Outport  Port=2  VectorParamsAs1DForOutWhenUnconnected=off
  wires:
  Demux/2 -> [t2]
  Demux/4 -> [t4]
  Demux/5 -> [t5]
  Demux/3 -> [t3]
  Demux/1 -> [t1]
  T/1 -> Demux/1
  Demux/6 -> [t6]
  [q6] -> Mux2/6
  [q4] -> Mux2/4
  [q3] -> Mux2/3
  [q5] -> Mux2/5
  [q2] -> Mux2/2
  [q1] -> Mux2/1
  Mux2/1 -> q/1
  [t1] -> Simulink-PS Converter/1
  PS-Simulink Converter/1 -> [q1]
  [t2] -> Simulink-PS Converter1/1
  PS-Simulink Converter1/1 -> [q2]
  [t3] -> Simulink-PS Converter2/1
  PS-Simulink Converter2/1 -> [q3]
  [t4] -> Simulink-PS Converter3/1
  PS-Simulink Converter3/1 -> [q4]
  [t5] -> Simulink-PS Converter4/1
  PS-Simulink Converter4/1 -> [q5]
  [t6] -> Simulink-PS Converter5/1
  PS-Simulink Converter5/1 -> [q6]
  [q11] -> Mux1/5
  Mux1/1 -> w/1
  [q9] -> Mux1/3
  [q8] -> Mux1/2
  [q10] -> Mux1/4
  [q7] -> Mux1/1
  [q12] -> Mux1/6
  PS-Simulink Converter6/1 -> [q7]
  PS-Simulink Converter7/1 -> [q8]
  PS-Simulink Converter8/1 -> [q9]
  PS-Simulink Converter9/1 -> [q10]
  PS-Simulink Converter10/1 -> [q11]
  PS-Simulink Converter11/1 -> [q12]
  connections:
  robot1_base/LConn1 -- base_link_base4/RConn1
  robot1_base/RConn1 -- joint_1/LConn1
  joint_5/LConn1 -- link_4/RConn1
  joint_3/RConn1 -- link_3/LConn1
  joint_2/RConn1 -- link_2/LConn1
  joint_3/LConn1 -- link_2/RConn1
  joint_1/RConn1 -- link_1/LConn1
  joint_4/RConn1 -- link_4/LConn1
  joint_4/LConn1 -- link_3/RConn1
  joint_5/RConn1 -- link_5/LConn1
  joint_2/LConn1 -- link_1/RConn1
  joint_6/RConn1 -- link_6/LConn1
  joint_6/LConn1 -- link_5/RConn1
  Robot1/RConn1 -- base_link_base4/LConn1
  In/RConn1 -- Robot1/LConn1
  joint6_tool2/LConn1 -- link_6/RConn1
  Out/RConn1 -- joint6_tool2/RConn1
  Simulink-PS Converter/RConn1 -- joint_1/LConn2
  joint_1/RConn2 -- PS-Simulink Converter/LConn1
  Simulink-PS Converter1/RConn1 -- joint_2/LConn2
  PS-Simulink Converter1/LConn1 -- joint_2/RConn2
  Simulink-PS Converter2/RConn1 -- joint_3/LConn2
  joint_3/RConn2 -- PS-Simulink Converter2/LConn1
  Simulink-PS Converter3/RConn1 -- joint_4/LConn2
  PS-Simulink Converter3/LConn1 -- joint_4/RConn2
  Simulink-PS Converter4/RConn1 -- joint_5/LConn2
  joint_5/RConn2 -- PS-Simulink Converter4/LConn1
  joint_6/RConn2 -- PS-Simulink Converter5/LConn1
  PS-Simulink Converter6/LConn1 -- joint_1/RConn3
  Simulink-PS Converter5/RConn1 -- joint_6/LConn2
  PS-Simulink Converter7/LConn1 -- joint_2/RConn3
  PS-Simulink Converter8/LConn1 -- joint_3/RConn3
  PS-Simulink Converter9/LConn1 -- joint_4/RConn3
  PS-Simulink Converter10/LConn1 -- joint_5/RConn3
  PS-Simulink Converter11/LConn1 -- joint_6/RConn3
